simulink model "MR_CIGRE_RESISTIVO"  (R2017b)
settings: Solver=ode23tb  StartTime=0.0  StopTime=t_sim  RelTol=1e-4
values from neighbouring files (symbols this model uses):
  Cdc_Bat1 = 2E-3    (= 0.002)    [Dados_de_Bat_1.m]
  Cf_Bat1 = 5E-6    (= 5e-06)    [Dados_de_Bat_1.m]
  I_max_Bat1 = 1.5*Is_bat1*sqrt(2)    [Dados_de_Bat_1.m]
  Is_bat1 = Sb_Bat1 / (sqrt(3)*Vs2)    [Dados_de_Bat_1.m]
  K_iff_Bat1 = 0    [Dados_de_Bat_1.m]
  Kcij = Rfsj*(2*sig*w_ij*(Tpj + Tfsj)-1)    (= 3.9715)    [Dados_de_Bat_1.m]
  Ki_Bat1 = (R_Bat1+ron_Bat1)/ti_Bat1    (= 201.76)    [Dados_de_Bat_1.m]
  Kp_Bat1 = L_Bat1/ti_Bat1    (= 2.7)    [Dados_de_Bat_1.m]
  Kv_Bat1 = 0.75    [Dados_de_Bat_1.m]
  Kvi_DC = 25*Kvp_DC    (= 7.5)    [Dados_de_Bat_1.m]
  Kvp_DC = 0.3    [Dados_de_Bat_1.m]
  L_10_18 = imag(ug3)*C_10_18    [Dados_de_Linhas.m]
  L_12_13 = imag(ug3)*C_12_13    [Dados_de_Linhas.m]
  L_13_14 = imag(ug3)*C_13_14    [Dados_de_Linhas.m]
  L_14_15 = imag(ug3)*C_14_15    [Dados_de_Linhas.m]
  L_1_2 = imag(ug1)*C_1_2    [Dados_de_Linhas.m]
  L_2_3 = imag(ug1)*C_2_3    [Dados_de_Linhas.m]
  L_3_11 = imag(ug3)*C_3_11    [Dados_de_Linhas.m]
  L_3_4 = imag(ug1)*C_3_4    [Dados_de_Linhas.m]
  L_4_12 = imag(ug3)*C_4_12    [Dados_de_Linhas.m]
  L_4_5 = imag(ug1)*C_4_5    [Dados_de_Linhas.m]
  L_5_6 = imag(ug1)*C_5_6    [Dados_de_Linhas.m]
  L_6_16 = imag(ug3)*C_6_16    [Dados_de_Linhas.m]
  L_6_7 = imag(ug1)*C_6_7    [Dados_de_Linhas.m]
  L_7_8 = imag(ug1)*C_7_8    [Dados_de_Linhas.m]
  L_8_9 = imag(ug1)*C_8_9    [Dados_de_Linhas.m]
  L_9_10 = imag(ug1)*C_9_10    [Dados_de_Linhas.m]
  L_9_17 = imag(ug3)*C_9_17    [Dados_de_Linhas.m]
  L_Bat1 = 1.35E-3    (= 0.00135)    [Dados_de_Bat_1.m]
  L_Bat2 = 1.35E-3    (= 0.00135)    [Dados_de_Bat_2.m]
  L_Virt_Bat1 = 3e-3    (= 0.003)    [Dados_de_Bat_1.m]
  L_Virt_Bat2 = 3.0E-3    (= 0.003)    [Dados_de_Bat_2.m]
  LC_Bat2 = 1e-16    [Dados_de_Bat_2.m]
  Lfsj = 4e-3    (= 0.004)    [Dados_de_Bat_1.m]
  LPF_Ci_Bat1 = 8000    [Dados_de_Bat_1.m]
  LPF_Ci_Bat2 = 5000    [Dados_de_Bat_2.m]
  LPF_Cv_Bat1 = 3000    [Dados_de_Bat_1.m]
  LPF_Q_Bat1 = 3*2*pi()    [Dados_de_Bat_1.m]
  m_Bat1 = 0.05    [Dados_de_Bat_1.m]
  n_Bat1 = 0.05    [Dados_de_Bat_1.m]
  PQ_ref_taxavar_bat1 = 0.5    [Dados_de_Bat_1.m]
  R_10_18 = real(ug3)*C_10_18    [Dados_de_Linhas.m]
  R_12_13 = real(ug3)*C_12_13    [Dados_de_Linhas.m]
  R_13_14 = real(ug3)*C_13_14    [Dados_de_Linhas.m]
  R_14_15 = real(ug3)*C_14_15    [Dados_de_Linhas.m]
  R_1_2 = real(ug1)*C_1_2    [Dados_de_Linhas.m]
  R_2_3 = real(ug1)*C_2_3    [Dados_de_Linhas.m]
  R_3_11 = real(ug3)*C_3_11    [Dados_de_Linhas.m]
  R_3_4 = real(ug1)*C_3_4    [Dados_de_Linhas.m]
  R_4_12 = real(ug3)*C_4_12    [Dados_de_Linhas.m]
  R_4_5 = real(ug1)*C_4_5    [Dados_de_Linhas.m]
  R_5_6 = real(ug1)*C_5_6    [Dados_de_Linhas.m]
  R_6_16 = real(ug3)*C_6_16    [Dados_de_Linhas.m]
  R_6_7 = real(ug1)*C_6_7    [Dados_de_Linhas.m]
  R_7_8 = real(ug1)*C_7_8    [Dados_de_Linhas.m]
  R_8_9 = real(ug1)*C_8_9    [Dados_de_Linhas.m]
  R_9_10 = real(ug1)*C_9_10    [Dados_de_Linhas.m]
  R_9_17 = real(ug3)*C_9_17    [Dados_de_Linhas.m]
  R_Bat1 = 0.1    [Dados_de_Bat_1.m]
  R_Virt_Bat1 = 0    [Dados_de_Bat_1.m]
  R_Virt_Bat2 = 0    [Dados_de_Bat_2.m]
  Rb_bat1 = (N_cell_serie * Rb_cell) / N_string_cell    (= 0.153333333333)    [Dados_de_Bat_1.m]
  RC_Bat2 = 1e-16    [Dados_de_Bat_2.m]
  Rfsj = 0.03    [Dados_de_Bat_1.m]
  ron_Bat1 = 0.88E-3    (= 0.00088)    [Dados_de_Bat_1.m]
  Vdc_Bat1 = 800    [Dados_de_Bat_1.m]
  Voc_bat1 = N_cell_serie * Voc_cell    (= 180)    [Dados_de_Bat_1.m]
  z_Bat1 = z_gk    [Dados_de_Bat_1.m]
undefined symbols (not defined in the file or in its folder): BAT1_CONT, BAT2_CONT, Cdc, Cf, cont_fre, cont_ten, f0, Imax_solar1, Imax_solar2, Ki_interm, Kie, Kiw, Kp_cp, Kp_cr, Kp_interm, Kpe, Kpw, L, LPF_P_Bat1, LPF_P_Interm, LPF_Vdc, P_Solar1, P_Solar2, PQ_ref_time_bat1, Pref_Bat1, Qref_Bat1, Qref_Solar, R, ron, Sb_Bat1, Sb_ger, Sb_sol1, Sb_sol2, t_atraso, t_CS_ini, TDR1, TDR11, TDR15, TDR16, TDR17, TDR18, ti_cp, ti_cr, tilha, TLR11, TLR15, TLR16, TLR17, TLR18, tsinc, Vdc, vref1, Vref_sec, Vs1, Vs2, w0, wref_sec
libraries: powerlib x158, powerlib_meascontrol x59, re_lib x2, simulink x1
(part 1 of 4)
Description:
  | Copyright 2008-2016 The MathWorks, Inc.
settings Model: FPTRunName=Active  SimulationMode=accelerator  ExtModeTrigMode=oneshot  ExtModeArmWhenConnect=off  ExtModeAutoUpdateStatusClock=off  Creator=MathWorks  LastModifiedBy=KDRF
settings SolverCC: ZeroCrossAlgorithm=Adaptive
settings DataIOCC: FinalStateName=MR_estab  InitialState=MR_estab  SaveCompleteFinalSimState=on  SaveFormat=Array  SignalLoggingSaveFormat=ModelDataLogs  SignalLoggingName=sigsOut  OutputTimes=[0:1/20:10]
settings OptimizationCC: BlockReduction=off  BooleanDataType=off  ExpressionDepthLimit=2147483647  InitFltsAndDblsToZero=on  EfficientMapNaN2IntZero=off  LifeSpan=inf
settings DebuggingCC: UnderspecifiedInitializationDetection=Classic  MergeDetectMultiDrivingBlocksExec=none  CheckExecutionContextPreStartOutputMsg=on  CheckExecutionContextRuntimeOutputMsg=on  SignalResolutionControl=TryResolveAllWithWarning  IgnoredZcDiagnostic=none  MultiTaskDSMMsg=warning  MultiTaskCondExecSysMsg=none  SigSpecEnsureSampleTimeMsg=none  FcnCallInpInsideContextMsg=warning  UnconnectedInputMsg=none  UnconnectedOutputMsg=none  UnconnectedLineMsg=none  StateNameClashWarn=warning  SFUnexpectedBacktrackingDiag=warning  SFNoUnconditionalDefaultTransitionDiag=warning  SFExecutionAtInitializationDiag=none
settings HardwareCC: ProdBitPerPointer=32  ProdBitPerSizeT=32  ProdBitPerPtrDiffT=32  ProdLargestAtomicFloat=None  ProdIntDivRoundTo=Undefined  ProdEndianess=Unspecified  ProdWordSize=32  ProdHWDeviceType=Specified  TargetBitPerPointer=64  TargetBitPerSizeT=64  TargetBitPerPtrDiffT=64  TargetLongLongMode=on  TargetIntDivRoundTo=Zero  TargetEndianess=LittleEndian  TargetWordSize=64  TargetHWDeviceType=MATLAB Host  ProdEqTarget=off
settings ModelReferenceCC: PropagateSignalLabelsOutOfModel=off
settings CodeAppCC: MaxIdLength=128
settings GRTTargetCC: TargetLangStandard=C89/C90 (ANSI)  CombineOutputUpdateFcns=off  GRTInterface=on
settings ConfigComp: CovMetricSettings=dw  CovHtmlReporting=on  CovSaveCumulativeToWorkspaceVar=on  CovSaveSingleToWorkspaceVar=on  CovExternalEMLEnable=off  CovSFcnEnable=off
settings SimscapeCC: SimscapeNormalizeSystem=off

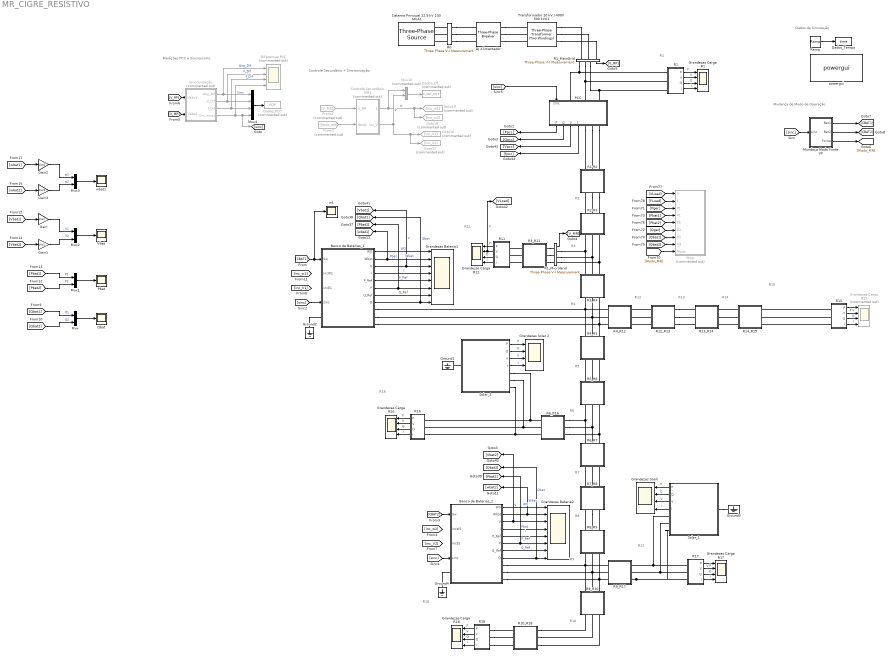
== system MR_CIGRE_RESISTIVO ==
  note: Medições PCC e Sincronismo
  note: Dados de Simulação
  note: R2
  note: R3
  note: R12
  note: R13
  note: R14
  note: R4
  note: R5
  note: R7
  note: R8
  note: R6
  note: R9
  note: R10
  note: R18
  note: R17
  note: R16
  note: R15
  note: R11
  note: R1
  note: Mudança de Modo de Operação
  note: Controle Secundário + Sincronização
  Banco de Baterias_1 : Subsystem
  Banco de Baterias_2 : Subsystem
  Controle Secundário MR1 : Subsystem  Commented=on
  "DJ Alimentador " : powerlib/Elements/Three-Phase Breaker  InitialState=closed  SwitchA=on  SwitchB=on  SwitchC=on  SwitchTimes=t_deslig_rede  External=off  BreakerResistance=0.01  SnubberResistance=1e5  SnubberCapacitance=inf  Measurements=None
      settings: AttributesFormatString=\n
  Dados_CS : ToWorkspace  Commented=on  VariableName=C_SEC_INC1  SaveFormat=Structure With Time  SampleTime=-1
  Dados_PCC : ToWorkspace  Commented=on  VariableName=PDF  SampleTime=-1
  Dados_Tempo : ToWorkspace  VariableName=time  SampleTime=-1
  Diferenças PCC : Scope  Commented=on  NumInputPorts=4
  From1 : From  Commented=on  GotoTag=Modo_MR
  From2 : From  Commented=on  GotoTag=V_MR
  Gain : Gain  Gain=1/Vs2
  Gain1 : Gain  Gain=1/Vs2
  Gain2 : Gain  Gain=1/w0
  Gain3 : Gain  Gain=1/w0
  Goto16 : Goto  Commented=on  GotoTag=inc_V1
  Goto17 : Goto  Commented=on  GotoTag=inc_V2
  Goto18 : Goto  Commented=on  GotoTag=inc_w2
  Goto19 : Goto  Commented=on  GotoTag=inc_w1
  Grandezas Bateria1 : Scope  NumInputPorts=8
  Grandezas Bateria2 : Scope  NumInputPorts=8
  Grandezas Carga R{1,11,16..18} (5 alike) : Scope  NumInputPorts=4
  Grandezas Carga R15 : Scope  Commented=on  NumInputPorts=4
  Grandezas Soalr : Scope  NumInputPorts=4
  Grandezas Solar 2 : Scope  NumInputPorts=4
  Ground{1..4} (4 alike) : powerlib/Elements/Ground  LConnTagsString=a
  Mundaça Modo Fonte VF : Subsystem
  Mux{,1..3} (4 alike) : Mux  Inputs=2
  Mux10 : Mux  Commented=on  Inputs=2
  Mux4 : Mux
  PCC : Subsystem
  Pbat : Scope
  Qbat : Scope
  R0 : powerlib/Measurements/Three-Phase V-I Measurement  VoltageMeasurement=phase-to-phase  SetLabelV=on  LabelV=V_sub  Vpu=off  VpuLL=off  CurrentMeasurement=no  SetLabelI=on  LabelI=Iabc_B120  Ipu=off  Pbase=100e6  Vbase=Vs1  OutputType=Complex  PhasorSimulation=on  PSBequivalent=0
  R1 : Subsystem
  R1-R2 : Subsystem
  R10_R18 : Subsystem
  R11 : Subsystem
  R12_R13 : Subsystem
  R13_R14 : Subsystem
  R14_R15 : Subsystem
  R15 : Subsystem
  R16 : Subsystem
  R17 : Subsystem
  R18 : Subsystem
  R1_MainGrid : powerlib/Measurements/Three-Phase V-I Measurement  VoltageMeasurement=phase-to-phase  SetLabelV=off  LabelV=Vabc_B120  Vpu=off  VpuLL=off  CurrentMeasurement=no  SetLabelI=off  LabelI=Iabc_B120  Ipu=off  Pbase=20e3  Vbase=Vs2  OutputType=Complex  PhasorSimulation=on  PSBequivalent=0
  R1_MicroGrid : powerlib/Measurements/Three-Phase V-I Measurement  VoltageMeasurement=phase-to-phase  SetLabelV=off  LabelV=Vabc_B120  Vpu=off  VpuLL=off  CurrentMeasurement=no  SetLabelI=off  LabelI=Iabc_B120  Ipu=off  Pbase=20e3  Vbase=Vs2  OutputType=Complex  PhasorSimulation=on  PSBequivalent=0
  R2-R3 : Subsystem
  R3_R11 : Subsystem
  R3_R4 : Subsystem
  R4_R12 : Subsystem
  R4_R5 : Subsystem
  R5_R6 : Subsystem
  R6_R16 : Subsystem
  R6_R7 : Subsystem
  R7_R8 : Subsystem
  R8_R9 : Subsystem
  R9_R10 : Subsystem
  R9_R17 : Subsystem
  Ramp : simulink/Sources/Ramp  slope=1  start=0  X0=0
  Sincronização : Subsystem  Commented=on
  Sistema Principal 22.9 kV 100 MVA1 : powerlib/Electrical Sources/Three-Phase Source  InternalConnection=Yg  VoltagePhases=off  Voltage=Vs1*vref1  PhaseAngle=0  Voltage_phases=[25e3 25e3 25e3]/sqrt(3)  PhaseAngles_phases=[0 -120 +120]  Frequency=f0  NonIdealSource=on  SpecifyImpedance=on  Resistance=25^2/1000/10  Inductance=25^2/1000/377  ShortCircuitLevel=100e6  BaseVoltage=Vs1  XRratio=1  BusType=swing  Pref=0  Qref=0  Prefabc=[10e3, 10e3, 10e3]  Qrefabc=[0, 0, 0]  Qmin=-Inf  Qmax=Inf
  Solar_1 : Subsystem
  Solar_2 : Subsystem
  Stop : Subsystem  Commented=on
  Transformador 20 kV / 400V 500 kVA1 : powerlib/Elements/Three-Phase Transformer (Two Windings)  Winding1Connection=Y  Winding2Connection=Yg  CoreType=Three single-phase transformers  SetSaturation=off  Hysteresis=off  DataFile='hysteresis'  SetInitialFlux=off  Measurements=None  UNITS=pu  NominalPower=[ 500e3 , 50 ]  Winding1=[Vs1 , 0.005 , 0.02]  Winding2=[Vs2 , 0.005 , 0.02 ]  Rm=200  Lm=200  L0=0.5  Saturation="[ 0,0  ;  0.005,1.2  ;  1.0,1.4 ]"  InitialFluxes=[ 0.8 , -0.8 , 0.7 ]  MoreParameters=off  BreakLoop=off  DataType=off  TransfoNumber=0
  Vbat : Scope
  powergui : powerlib/powergui  Priority=2  SimulationMode=Discrete  SampleTime=10e-6  frequency=60  Iterations=50  frequencyindice=0  Pbase=20e3  ErrMax=0.0001  UnitsV=V  UnitsW=kW  buscounter=0  FunctionMessages=off  echomessages=off  EnableUseOfTLC=off  CurrentSourceSwitches=off  DisableSnubberDevices=on  DisableRonSwitches=off  DisableVfSwitches=off  DisplayEquations=off  SolverType=Tustin  Interpol=off  ExternalGateDelay=off  methode=off  Ts=0  x0status=blocks  SPID=on  SwTol=0  HookPort=off  RestoreLinks=warning  ResistiveCurrentMeasurement=off  Frange=logspace(0,3,50)  Ylog=off  Xlog=off  ShowGrid=off  save=off  variable=ZData  structure=0  ZoomFFT=on  StartTime=0.0  cycles=2  DisplayStyle=off  fundamental=60  FreqAxis=off  MaxFrequency=1000  frequencyindicesteady=1  RmsSteady=1  display=off
  w1 : Scope
  wbat1 : Scope
  wires:
  Mux4/1 -> Dados_PCC/1
  Ramp/1 -> Dados_Tempo/1
  [V_MR] -> Sincronização/2(Vabc2)
  [V_RP] -> Sincronização/1(Vabc1)
  Sincronização/1(Ang_Dif) -> Diferenças PCC/1, Mux4/1  "Ang_Dif"
  Sincronização/2(V_Dif) -> Diferenças PCC/2, Mux4/2  "V_Dif"
  Sincronização/3(f_Dif) -> Diferenças PCC/3, Mux4/3  "f_Dif"
  Sincronização/4(Sinal sinc1) -> Diferenças PCC/4, [sinc], Mux4/4  "Sinc"
  Solar_2/1(P) -> Grandezas Solar 2/1  "P"
  Solar_2/2(Q) -> Grandezas Solar 2/2  "Q"
  Solar_2/3(V) -> Grandezas Solar 2/3  "V"
  Solar_2/4(I) -> Grandezas Solar 2/4  "I"
  Solar_1/1(P) -> Grandezas Soalr/1  "P"
  Solar_1/2(Q) -> Grandezas Soalr/2  "Q"
  Solar_1/3(V) -> Grandezas Soalr/3  "V"
  Solar_1/4(I) -> Grandezas Soalr/4  "I"
  R1_MainGrid/1 -> [V_RP]
  Banco de Baterias_1/2(Wbat) -> [wbat1], Grandezas Bateria1/2  "Wbat"
  Banco de Baterias_1/4(I) -> Grandezas Bateria1/4  "I"
  Banco de Baterias_1/7(Q_Ref) -> Grandezas Bateria1/7  "Q_Ref"
  Banco de Baterias_1/5(P_Ref) -> Grandezas Bateria1/5  "P_Ref"
  Banco de Baterias_1/3(V) -> [Vbat1], Grandezas Bateria1/3  "V"
  [CBAT1] -> w1/1, Banco de Baterias_1/1(Sw)
  Banco de Baterias_1/6(P) -> [Pbat1], Grandezas Bateria1/6  "Pbat"
  Banco de Baterias_1/8(Q) -> [Qbat1], Grandezas Bateria1/8  "Qbat"
  [sinc] -> Banco de Baterias_1/4(sinc)
  Banco de Baterias_1/1(W0) -> Grandezas Bateria1/1  "W0"
  Banco de Baterias_2/7(Q_Ref) -> Grandezas Bateria2/7  "Q_Ref"
  Banco de Baterias_2/6(P) -> [Pbat2], Grandezas Bateria2/6  "Pbat"
  Banco de Baterias_2/4(I) -> Grandezas Bateria2/4  "I"
  Banco de Baterias_2/8(Q) -> [Qbat2], Grandezas Bateria2/8  "Qbat"
  Banco de Baterias_2/3(V) -> [Vbat2], Grandezas Bateria2/3  "V"
  Banco de Baterias_2/1(W0) -> Grandezas Bateria2/1  "W0"
  [sinc] -> Banco de Baterias_2/4(sinc)
  [CBAT2] -> Banco de Baterias_2/1(Sw)
  Banco de Baterias_2/2(Wbat) -> [wbat2], Grandezas Bateria2/2  "Wbat"
  Banco de Baterias_2/5(P_Ref) -> Grandezas Bateria2/5  "P_Ref"
  R1_MicroGrid/1 -> [V_MR]
  [Pbat1] -> Stop/4(P2)
  [VLoad] -> Stop/1(V)
  [Qger] -> Stop/6(Q1)
  [Modo_MR] -> Stop/9(Modo)
  [Qbat1] -> Stop/7(Q2)
  [Pger] -> Stop/3(P1)
  [Qbat2] -> Stop/8(Q3)
  [FLoad] -> Stop/2(f)
  [Pbat2] -> Stop/5(P3)
  R11/1(P) -> Grandezas Carga R11/1  "P"
  R11/2(V) -> [VLoad], Grandezas Carga R11/2  "V"
  R11/3(Q) -> Grandezas Carga R11/3  "Q"
  R11/4(I) -> Grandezas Carga R11/4  "I"
  R15/3(Q) -> Grandezas Carga R15/3  "Q"
  R15/2(V) -> Grandezas Carga R15/2  "V"
  R15/4(I) -> Grandezas Carga R15/4  "I"
  R15/1(P) -> Grandezas Carga R15/1  "P"
  R16/4(I) -> Grandezas Carga R16/4  "I"
  R16/3(Q) -> Grandezas Carga R16/3  "Q"
  R16/2(V) -> Grandezas Carga R16/2  "V"
  R16/1(P) -> Grandezas Carga R16/1  "P"
  R17/1(P) -> Grandezas Carga R17/1  "P"
  R17/3(Q) -> Grandezas Carga R17/3  "Q"
  R17/4(I) -> Grandezas Carga R17/4  "I"
  R17/2(V) -> Grandezas Carga R17/2  "V"
  R18/3(Q) -> Grandezas Carga R18/3  "Q"
  R18/2(V) -> Grandezas Carga R18/2  "V"
  R18/4(I) -> Grandezas Carga R18/4  "I"
  R18/1(P) -> Grandezas Carga R18/1  "P"
  R1/2(V) -> Grandezas Carga R1/2  "V"
  R1/4(I) -> Grandezas Carga R1/4  "I"
  R1/3(Q) -> Grandezas Carga R1/3  "Q"
  R1/1(P) -> Grandezas Carga R1/1  "P"
  PCC/4(f) -> [fpcc]
  PCC/3(V) -> [Vpcc]
  PCC/2(Q) -> [Qpcc]
  PCC/1(P) -> [Ppcc]
  [sinc] -> PCC/1(sinc)
  Mundaça Modo Fonte VF/1(Bat1) -> [CBAT1]
  Mundaça Modo Fonte VF/3(Fonte) -> [Modo_MR]
  Mundaça Modo Fonte VF/2(Bat2) -> [CBAT2]
  [sinc] -> Mundaça Modo Fonte VF/1(sinc)
  Controle Secundário MR1/1(Inc_w) -> Goto18/1, Goto19/1, Mux10/1  "w"
  Mux10/1 -> Dados_CS/1
  From2/1 -> Controle Secundário MR1/1(V_MR)
  From1/1 -> Controle Secundário MR1/2(Modo)
  Controle Secundário MR1/2(Inc_V) -> Goto17/1, Goto16/1, Mux10/2  "V"
  Mux/1 -> Qbat/1
  [Qbat1] -> Mux/1  "Q1"
  [Qbat2] -> Mux/2  "Q2"
  [Pbat1] -> Mux1/1  "P1"
  Mux1/1 -> Pbat/1
  [Pbat2] -> Mux1/2  "P2"
  [Vbat2] -> Gain1/1
  Mux2/1 -> Vbat/1
  [Vbat1] -> Gain/1
  Gain/1 -> Mux2/1  "V1"
  Gain1/1 -> Mux2/2  "V2"
  Mux3/1 -> wbat1/1
  Gain2/1 -> Mux3/1  "w1"
  [wbat1] -> Gain2/1
  Gain3/1 -> Mux3/2  "w2"
  [wbat2] -> Gain3/1
  connections:
  Solar_2/LConn1 -- Ground1/LConn1
  Solar_1/LConn1 -- Ground3/LConn1
  R3_R4/RConn1 -- R1_MicroGrid/RConn1 -- R2-R3/RConn1
  R3_R4/RConn2 -- R1_MicroGrid/RConn2 -- R2-R3/RConn2
  R3_R4/RConn3 -- R1_MicroGrid/RConn3 -- R2-R3/RConn3
  R12_R13/LConn1 -- R4_R12/RConn1
  R12_R13/LConn2 -- R4_R12/RConn2
  R12_R13/LConn3 -- R4_R12/RConn3
  R4_R12/LConn1 -- Banco de Baterias_1/RConn1 -- R4_R5/LConn1 -- R3_R4/LConn1
  R4_R12/LConn2 -- Banco de Baterias_1/RConn2 -- R4_R5/LConn2 -- R3_R4/LConn2
  R4_R12/LConn3 -- Banco de Baterias_1/RConn3 -- R4_R5/LConn3 -- R3_R4/LConn3
  R14_R15/LConn3 -- R13_R14/RConn3
  R14_R15/LConn1 -- R13_R14/RConn1
  R14_R15/LConn2 -- R13_R14/RConn2
  R12_R13/RConn1 -- R13_R14/LConn1
  R12_R13/RConn2 -- R13_R14/LConn2
  R12_R13/RConn3 -- R13_R14/LConn3
  R15/LConn1 -- R14_R15/RConn1
  R15/LConn2 -- R14_R15/RConn2
  R15/LConn3 -- R14_R15/RConn3
  R5_R6/LConn1 -- R4_R5/RConn1
  R5_R6/LConn2 -- R4_R5/RConn2
  R5_R6/LConn3 -- R4_R5/RConn3
  R16/LConn1 -- Solar_2/RConn1 -- R6_R16/RConn1
  R16/LConn3 -- Solar_2/RConn3 -- R6_R16/RConn3
  R16/LConn2 -- Solar_2/RConn2 -- R6_R16/RConn2
  R6_R16/LConn1 -- R6_R7/LConn1 -- R5_R6/RConn1
  R6_R16/LConn2 -- R6_R7/LConn2 -- R5_R6/RConn2
  R6_R16/LConn3 -- R6_R7/LConn3 -- R5_R6/RConn3
  R7_R8/LConn2 -- R6_R7/RConn2
  R7_R8/LConn1 -- R6_R7/RConn1
  R7_R8/LConn3 -- R6_R7/RConn3
  R8_R9/LConn1 -- R7_R8/RConn1
  R8_R9/LConn3 -- R7_R8/RConn3
  R7_R8/RConn2 -- R8_R9/LConn2
  R17/LConn1 -- Solar_1/RConn1 -- R9_R17/RConn1
  R17/LConn2 -- Solar_1/RConn2 -- R9_R17/RConn2
  R9_R17/RConn3 -- Solar_1/RConn3 -- R17/LConn3
  R9_R17/LConn1 -- Banco de Baterias_2/RConn1 -- R9_R10/LConn1 -- R8_R9/RConn1
  R9_R17/LConn2 -- Banco de Baterias_2/RConn2 -- R9_R10/LConn2 -- R8_R9/RConn2
  R9_R17/LConn3 -- Banco de Baterias_2/RConn3 -- R9_R10/LConn3 -- R8_R9/RConn3
  R10_R18/LConn1 -- R9_R10/RConn1
  R10_R18/LConn2 -- R9_R10/RConn2
  R10_R18/LConn3 -- R9_R10/RConn3
  R0/RConn1 -- Sistema Principal 22.9 kV 100 MVA1/RConn3
  R0/RConn2 -- Sistema Principal 22.9 kV 100 MVA1/RConn2
  R0/RConn3 -- Sistema Principal 22.9 kV 100 MVA1/RConn1
  R0/LConn1 -- "DJ Alimentador "/RConn3
  R0/LConn2 -- "DJ Alimentador "/RConn2
  R0/LConn3 -- "DJ Alimentador "/RConn1
  Transformador 20 kV / 400V 500 kVA1/RConn1 -- R1_MainGrid/LConn3
  Transformador 20 kV / 400V 500 kVA1/RConn2 -- R1_MainGrid/LConn2
  Transformador 20 kV / 400V 500 kVA1/RConn3 -- R1_MainGrid/LConn1
  PCC/RConn1 -- R1-R2/LConn1
  R1-R2/RConn1 -- R2-R3/LConn1
  R1-R2/RConn2 -- R2-R3/LConn2
  R1-R2/RConn3 -- R2-R3/LConn3
  Banco de Baterias_1/LConn1 -- Ground2/LConn1
  Banco de Baterias_2/LConn1 -- Ground4/LConn1
  R3_R11/LConn1 -- R1_MicroGrid/LConn1
  R3_R11/LConn2 -- R1_MicroGrid/LConn2
  R3_R11/LConn3 -- R1_MicroGrid/LConn3
  R3_R11/RConn1 -- R11/LConn1
  R3_R11/RConn3 -- R11/LConn3
  R3_R11/RConn2 -- R11/LConn2
  R18/LConn1 -- R10_R18/RConn1
  R18/LConn2 -- R10_R18/RConn2
  R18/LConn3 -- R10_R18/RConn3
  PCC/RConn2 -- R1-R2/LConn2
  PCC/RConn3 -- R1-R2/LConn3
  R1_MainGrid/RConn2 -- R1/LConn2 -- PCC/LConn2
  R1_MainGrid/RConn3 -- R1/LConn1 -- PCC/LConn1
  R1_MainGrid/RConn1 -- R1/LConn3 -- PCC/LConn3
  "DJ Alimentador "/LConn1 -- Transformador 20 kV / 400V 500 kVA1/LConn1
  "DJ Alimentador "/LConn2 -- Transformador 20 kV / 400V 500 kVA1/LConn2
  "DJ Alimentador "/LConn3 -- Transformador 20 kV / 400V 500 kVA1/LConn3

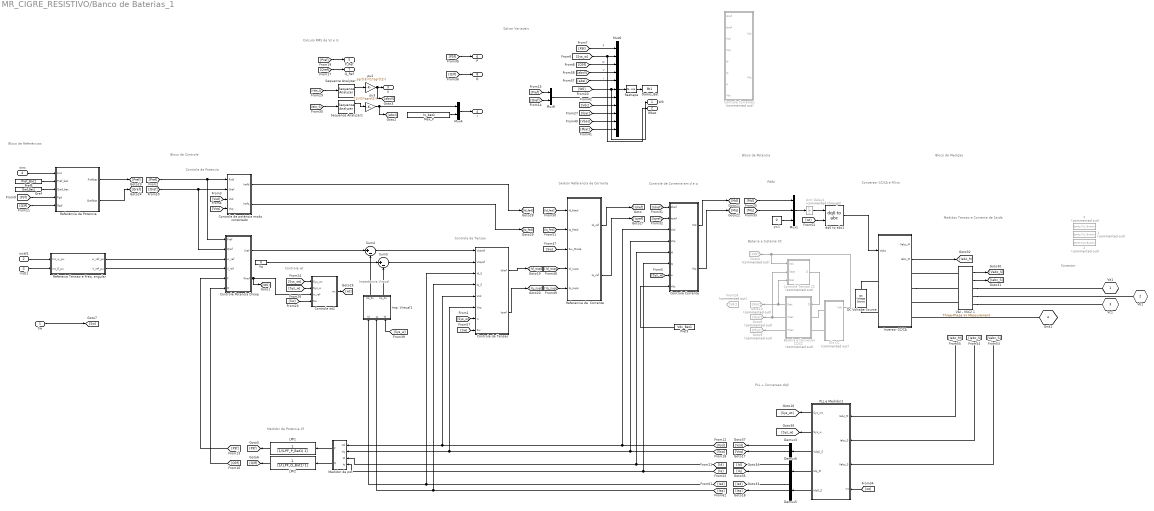
== system MR_CIGRE_RESISTIVO/Banco de Baterias_1 ==
  note: Bloco de Controle
  note: Controle de Corrente
      | em d e q
  note: Calculo RMS de Vs e Is
  note: Medidor de Potência 3f
  note: Seletor Referencia
      |      de Corrente
  note: Controle de Tensao
  note: Impedancia
      | 					  Virtual
  note: PWM
  note: Conversor CC/CA
      |           e Filtro
  note: Bloco de Potencia
  note: Bloco de Mediçao
  note: Medidas Tensao e
      |    Corrente de Saida
  note: PLL + Conversao dq0
  note: Bloco de Referências
  note: Controle de Potencia
  note: Controle wt
  note: Conector
  note: Bateria e Sistema CC
  note: Salvar Variaveis
  Sw : Inport
  incW1 : Inport  Port=2
  incE1 : Inport  Port=3
  sinc : Inport  Port=4
  1 : powerlib/Elements/Series RLC Branch  Commented=on  LConnTagsString=__new0  RConnTagsString=__new0  BranchType=RL  Resistance=RC_Bat2  Inductance=LC_Bat2  SetiL0=off  InitialCurrent=0  Capacitance=1e-6  Setx0=off  InitialVoltage=0  Measurements=None
  2 : powerlib/Elements/Series RLC Branch  Commented=on  LConnTagsString=__new0  RConnTagsString=__new0  BranchType=RL  Resistance=RC_Bat2  Inductance=LC_Bat2  SetiL0=off  InitialCurrent=0  Capacitance=1e-6  Setx0=off  InitialVoltage=0  Measurements=None
  9 : powerlib/Elements/Series RLC Branch  Commented=on  LConnTagsString=__new0  RConnTagsString=__new0  BranchType=RL  Resistance=RC_Bat2  Inductance=LC_Bat2  SetiL0=off  InitialCurrent=0  Capacitance=1e-6  Setx0=off  InitialVoltage=0  Measurements=None
  Bateria e Conversor CC/CC : Subsystem  Commented=on
  Controle Corrente : Subsystem
  Controle Corrente1 : Subsystem  Commented=on
  Controle Tensao CC : Subsystem  Commented=on
  Controle Potencia Droop : Subsystem
  Controle de Tensao : Subsystem
  Controle de potência modo conectado : Subsystem
  Controle wt2 : Subsystem
  DC Voltage Source : powerlib/Electrical Sources/DC Voltage Source  Amplitude=Vdc_Bat1  Measurements=None
  Dados_Bat : ToWorkspace  VariableName=Bt1  SaveFormat=Structure With Time  SampleTime=-1
  Demux3 : Demux  Outputs=3
  Demux5 : Demux  Outputs=3
  Demux6 : Demux  Outputs=3
  Elo CC : Subsystem  Commented=on
  From28 : From  Commented=on  GotoTag=Vdc
  Goto10 : Goto  Commented=on  GotoTag=Ibat
  Goto4 : Goto  Commented=on  GotoTag=Vdc
  Goto8 : Goto  Commented=on  GotoTag=Vbat
  Goto9 : Goto  Commented=on  GotoTag=Pbat
  Imp. Virtual1 : Subsystem
  Inversor CC/CA : Subsystem
  LPF1 : TransferFcn  Denominator=[1/(LPF_P_Bat1) 1]
  LPF2 : TransferFcn  Denominator=[1/(LPF_Q_Bat1) 1]
  Max_P : Constant  Value=Is_bat1
  Medidor de pot : Subsystem
  Mux1 : Mux  Inputs=3
  Mux4 : Mux  Inputs=2
  Mux6 : Mux  Inputs=11
  Mux8 : Mux  Inputs=2
  PLL e Medidor1 : Subsystem
  Pref3 : Constant  Value=Vdc_Bat1
  Pref5 : Constant  Value=Pref_Bat1
  Qref : Constant  Value=Qref_Bat1
  Referecia Tensao e Freq. angular : Subsystem
  Referencia de  Corrente : Subsystem
  Referência de Potencia : Subsystem
  Reshape : Reshape  OutputDimensions=[1,7]
  Sequence Analyzer : powerlib_meascontrol/Measurements/Sequence Analyzer  Freq=f0  n=1  seq=Positive  InInit=[1, 0]  Ts=0
      settings: SourceProductName=Simscape Power Systems  SourceProductBaseCode=PS
  Sequence Analyzer1 : powerlib_meascontrol/Measurements/Sequence Analyzer  Freq=f0  n=1  seq=Positive  InInit=[1, 0]  Ts=0
      settings: SourceProductName=Simscape Power Systems  SourceProductBaseCode=PS
  Sum4 : Sum  Inputs=|+-
  Sum5 : Sum  Inputs=|+-
  Unit Delay1 : UnitDelay  Commented=through  SampleTime=5E-6
  V&I - VSC2 1 : powerlib/Measurements/Three-Phase V-I Measurement  VoltageMeasurement=phase-to-ground  SetLabelV=off  LabelV=Vabc  Vpu=off  VpuLL=off  CurrentMeasurement=yes  SetLabelI=off  LabelI=Iabc  Ipu=off  Pbase=100e6  Vbase=500e3  OutputType=Complex  PhasorSimulation=off  PSBequivalent=0
  Vq : Constant  Value=0
  dq0 to abc1 : powerlib_meascontrol/Transformations/dq0 to abc  Alignment=90 degrees behind phase A axis
  pu2 : Gain  Gain=sqrt(3)/(1*sqrt(2))
  pu3 : Gain  Gain=(1)/(1*sqrt(2))
  y=1 : Constant  Value=0
  Va1 : PMIOPort  Port=1  Side=Right
  Vb1 : PMIOPort  Port=2  Side=Right
  Vc1 : PMIOPort  Port=3  Side=Right
  Gnd1 : PMIOPort  Port=4  Side=Left
  W0 : Outport
  Wbat : Outport  Port=2
  V : Outport  Port=3
  I : Outport  Port=4
  P_Ref : Outport  Port=5
  P : Outport  Port=6
  Q_Ref : Outport  Port=7
  Q : Outport  Port=8
  wires:
  Sequence Analyzer/1 -> pu2/1
  pu2/1 -> [absV], V/1
  Sequence Analyzer1/1 -> pu3/1
  [Vabc_S] -> Sequence Analyzer/1
  [Iabc_S] -> Sequence Analyzer1/1
  [Sys_w] -> Controle Corrente/7(w)
  [Iq] -> Medidor de pot/4(Iq), Controle Corrente/6(Iq)
  [Idref] -> Controle Corrente/1(Idref)
  [Iqref] -> Controle Corrente/2(Iqref)
  Controle Corrente/1(Md) -> [Md]
  Mux4/1 -> I/1
  pu3/1 -> Mux4/1, [absI]
  [Q3f] -> Q/1
  Max_P/1 -> Mux4/2
  Referencia de  Corrente/1(Id_ref) -> [Idref]
  [Sw] -> Referencia de  Corrente/3(Sw_Mode)
  Controle de Tensao/1(Idref) -> [Id_sup]
  Controle de Tensao/2(Iqref) -> [Iq_sup]
  [Iq_sup] -> Referencia de  Corrente/5(Iq_supp)
  [Id_fed] -> Referencia de  Corrente/1(Id_feed)
  [Iq_fed] -> Referencia de  Corrente/2(Iq_feed)
  Controle de potência modo conectado/1(Irefd) -> [Id_fed]
  Controle de potência modo conectado/2(Irefq) -> [Iq_fed]
  [Mq] -> Mux1/2
  [Md] -> Mux1/1
  V&I - VSC2 1/2 -> [Iabc_S]
  V&I - VSC2 1/1 -> [Vabc_S]
  Mux1/1 -> Unit Delay1/1
  y=1/1 -> Mux1/3
  Inversor CC/CA/2(Iabc_M) -> [Iabc_M]
  Sum4/1 -> Controle de Tensao/1(Vsdref)
  Sum5/1 -> Controle de Tensao/2(Vsqref)
  Demux6/1 -> [Id]
  [wt] -> PLL e Medidor1/4(wt)
  PLL e Medidor1/5(Idq0_S) -> Demux5/1
  PLL e Medidor1/4(Idq_M) -> Demux6/1
  PLL e Medidor1/3(Vdq0_S) -> Demux3/1
  Demux5/1 -> [Isd]
  Demux6/2 -> [Iq]
  PLL e Medidor1/2(Sys_w) -> [Sys_w]
  Demux3/1 -> [Vsd]
  PLL e Medidor1/1(Sys_wt) -> [Sys_wt]
  Demux5/2 -> [Isq]
  Demux3/2 -> [Vsq]
  [Sw] -> Controle de Tensao/8(Sw)
  [Sys_w] -> Controle de Tensao/7(w)
  [Isq] -> Controle de Tensao/4(Iq_S), Imp. Virtual1/2(Iq)
  [Isd] -> Controle de Tensao/3(Id_S), Imp. Virtual1/1(Id)
  Sw/1 -> [Sw]
  Referência de Potencia/2(Qrefbat) -> [Qref]
  incE1/1 -> Referecia Tensao e Freq. angular/2(Inc_E_pu)
  Pref5/1 -> Referência de Potencia/2(Pref_bat)
  [P3f] -> Referência de Potencia/4(Pgd)
  Qref/1 -> Referência de Potencia/3(Qref_bat)
  [Q3f] -> Referência de Potencia/5(Qgd)
  Referência de Potencia/1(Prefbat) -> [Pref]
  sinc/1 -> Referência de Potencia/1(sinc)
  incW1/1 -> Referecia Tensao e Freq. angular/1(Inc_w_pu)
  [Pref] -> Controle Potencia Droop/1(Pref), Controle de potência modo conectado/1(Pref)
  [Qref] -> Controle Potencia Droop/2(Qref), Controle de potência modo conectado/2(Qref)
  Referecia Tensao e Freq. angular/1(w_ref_pu) -> Controle Potencia Droop/3(w_ref)
  Referecia Tensao e Freq. angular/2(V_ref_pu) -> Controle Potencia Droop/4(V_ref)
  [P3f] -> Controle Potencia Droop/5(P)
  [Q3f] -> Controle Potencia Droop/6(Q)
  Vq/1 -> Sum5/1
  [Pref] -> P_Ref/1
  [Qref] -> Q_Ref/1
  [P3f] -> P/1
  [Sys_w] -> Imp. Virtual1/3(W)
  [Sw] -> Controle wt2/4(Sw)
  [Sys_wt] -> Controle wt2/1(Sys_wt)
  Controle Potencia Droop/2(Wref) -> Controle wt2/3(w_ref), [W0]
  [Vsd] -> Controle de potência modo conectado/3(Vsd)
  [Vsq] -> Controle de potência modo conectado/4(Vsq)
  [Sys_w] -> Controle wt2/2(Sys_w)
  LPF1/1 -> [P3f]
  LPF2/1 -> [Q3f]
  Medidor de pot/2(Q) -> LPF2/1
  [Iabc_M] -> PLL e Medidor1/1(Iabc_M)
  [Iabc_S] -> PLL e Medidor1/2(Iabc_S)
  Controle Potencia Droop/1(Vref) -> Sum4/1
  Imp. Virtual1/1(Vd_Zv) -> Sum4/2
  Imp. Virtual1/2(Vq_Zv) -> Sum5/2
  Controle wt2/1(wt) -> [wt]
  [wt] -> dq0 to abc1/2
  dq0 to abc1/1 -> Inversor CC/CA/1(Vabc)
  Referencia de  Corrente/2(Iq_ref) -> [Iqref]
  [Id_sup] -> Referencia de  Corrente/4(Id_supp)
  [Id] -> Medidor de pot/3(Id), Controle Corrente/5(Id)
  [Vabc_S] -> PLL e Medidor1/3(Vabc_S)
  [Vsd] -> Controle de Tensao/5(Vsd), Medidor de pot/1(Vd), Controle Corrente/3(Vsd)
  [Vsq] -> Medidor de pot/2(Vq), Controle de Tensao/6(Vsq), Controle Corrente/4(Vsq)
  Controle Corrente/2(Mq) -> [Mq]
  Medidor de pot/1(P) -> LPF1/1
  Bateria e Conversor CC/CC/1(Ibat) -> Goto10/1, Controle Tensao CC/3(Ibat)
  Controle Tensao CC/1(D) -> Bateria e Conversor CC/CC/1(D)
  Bateria e Conversor CC/CC/3(Pbat) -> Goto9/1
  Bateria e Conversor CC/CC/2(Vbat) -> Goto8/1, Controle Tensao CC/2(Vbat)
  Elo CC/1(Vdc) -> Controle Tensao CC/1(Vdc), Goto4/1
  [Q3f] -> Mux6/3  "Q"
  [W0] -> W0/1, Mux6/6
  Mux8/1 -> Mux6/7
  Mux6/1 -> Reshape/1
  Reshape/1 -> Dados_Bat/1
  [absV] -> Mux6/4  "V"
  [Pbat] -> Mux6/11
  [P3f] -> Mux6/1  "P"
  [absI] -> Mux6/5  "I"
  [Vbat] -> Mux6/10
  [Vdc] -> Mux6/8
  [Pref] -> Mux8/1
  [Sys_w] -> Wbat/1, Mux6/2
  [Qref] -> Mux8/2
  [Ibat] -> Mux6/9
  Unit Delay1/1 -> dq0 to abc1/1
  Pref3/1 -> Controle Corrente/8(Vdc)
  connections:
  Gnd1/RConn1 -- Inversor CC/CA/RConn4
  V&I - VSC2 1/RConn3 -- Vc1/RConn1
  Inversor CC/CA/RConn2 -- V&I - VSC2 1/LConn2
  V&I - VSC2 1/RConn1 -- Va1/RConn1
  V&I - VSC2 1/LConn1 -- Inversor CC/CA/RConn1
  V&I - VSC2 1/LConn3 -- Inversor CC/CA/RConn3
  V&I - VSC2 1/RConn2 -- Vb1/RConn1
  Elo CC/LConn1 -- Bateria e Conversor CC/CC/LConn1
  Elo CC/LConn2 -- Bateria e Conversor CC/CC/LConn2
  DC Voltage Source/RConn1 -- Inversor CC/CA/LConn1
  DC Voltage Source/LConn1 -- Inversor CC/CA/LConn2

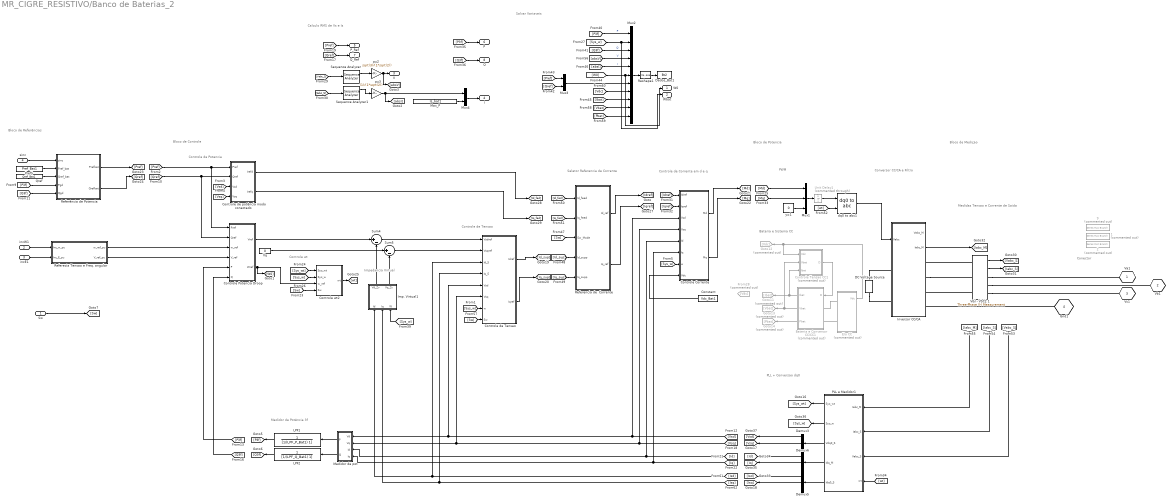
== system MR_CIGRE_RESISTIVO/Banco de Baterias_2 ==
  note: Bloco de Controle
  note: Controle de Corrente
      | em d e q
  note: Calculo RMS de Vs e Is
  note: Medidor de Potência 3f
  note: Seletor Referencia
      |      de Corrente
  note: Controle de Tensao
  note: Impedancia
      | 					  Virtual
  note: PWM
  note: Conversor CC/CA
      |           e Filtro
  note: Bloco de Potencia
  note: Bloco de Mediçao
  note: Medidas Tensao e
      |    Corrente de Saida
  note: PLL + Conversao dq0
  note: Bloco de Referências
  note: Controle de Potencia
  note: Controle wt
  note: Conector
  note: Salvar Variaveis
  note: Bateria e Sistema CC
  Sw : Inport
  incW1 : Inport  Port=2
  incE1 : Inport  Port=3
  sinc : Inport  Port=4
  1 : powerlib/Elements/Series RLC Branch  Commented=on  LConnTagsString=__new0  RConnTagsString=__new0  BranchType=RL  Resistance=RC_Bat2  Inductance=LC_Bat2  SetiL0=off  InitialCurrent=0  Capacitance=1e-6  Setx0=off  InitialVoltage=0  Measurements=None
  2 : powerlib/Elements/Series RLC Branch  Commented=on  LConnTagsString=__new0  RConnTagsString=__new0  BranchType=RL  Resistance=RC_Bat2  Inductance=LC_Bat2  SetiL0=off  InitialCurrent=0  Capacitance=1e-6  Setx0=off  InitialVoltage=0  Measurements=None
  9 : powerlib/Elements/Series RLC Branch  Commented=on  LConnTagsString=__new0  RConnTagsString=__new0  BranchType=RL  Resistance=RC_Bat2  Inductance=LC_Bat2  SetiL0=off  InitialCurrent=0  Capacitance=1e-6  Setx0=off  InitialVoltage=0  Measurements=None
  Bateria e Conversor CC/CC1 : Subsystem  Commented=on
  Constant : Constant  Value=Vdc_Bat1
  Controle Corrente : Subsystem
  Controle Tensao CC1 : Subsystem  Commented=on
  Controle Potencia Droop : Subsystem
  Controle de Tensao : Subsystem
  Controle de potência modo conectado : Subsystem
  Controle wt2 : Subsystem
  DC Voltage Source : powerlib/Electrical Sources/DC Voltage Source  Amplitude=Vdc_Bat1  Measurements=None
  Dados_Bat1 : ToWorkspace  VariableName=Bt2  SaveFormat=Structure With Time  SampleTime=-1
  Demux3 : Demux  Outputs=3
  Demux5 : Demux  Outputs=3
  Demux6 : Demux  Outputs=3
  Elo CC : Subsystem  Commented=on
  From28 : From  Commented=on  GotoTag=Vdc
  Goto11 : Goto  Commented=on  GotoTag=Ibat
  Goto12 : Goto  Commented=on  GotoTag=Vdc
  Goto13 : Goto  Commented=on  GotoTag=Vbat
  Goto14 : Goto  Commented=on  GotoTag=Pbat
  Imp. Virtual1 : Subsystem
  Inversor CC/CA : Subsystem
  LPF1 : TransferFcn  Denominator=[1/(LPF_P_Bat1) 1]
  LPF2 : TransferFcn  Denominator=[1/(LPF_Q_Bat1) 1]
  Max_P : Constant  Value=Is_bat1
  Medidor de pot : Subsystem
  Mux1 : Mux  Inputs=3
  Mux2 : Mux  Inputs=11
  Mux3 : Mux  Inputs=2
  Mux4 : Mux  Inputs=2
  PLL e Medidor1 : Subsystem
  Pref5 : Constant  Value=Pref_Bat1
  Qref : Constant  Value=Qref_Bat1
  Referecia Tensao e Freq. angular : Subsystem
  Referencia de  Corrente : Subsystem
  Referência de Potencia : Subsystem
  Reshape1 : Reshape  OutputDimensions=[1,7]
  Sequence Analyzer : powerlib_meascontrol/Measurements/Sequence Analyzer  Freq=f0  n=1  seq=Positive  InInit=[1, 0]  Ts=0
      settings: SourceProductName=Simscape Power Systems  SourceProductBaseCode=PS
  Sequence Analyzer1 : powerlib_meascontrol/Measurements/Sequence Analyzer  Freq=f0  n=1  seq=Positive  InInit=[1, 0]  Ts=0
      settings: SourceProductName=Simscape Power Systems  SourceProductBaseCode=PS
  Sum4 : Sum  Inputs=|+-
  Sum5 : Sum  Inputs=|+-
  Unit Delay1 : UnitDelay  Commented=through  SampleTime=5E-6
  V&I - VSC2 1 : powerlib/Measurements/Three-Phase V-I Measurement  VoltageMeasurement=phase-to-ground  SetLabelV=off  LabelV=Vabc  Vpu=off  VpuLL=off  CurrentMeasurement=yes  SetLabelI=off  LabelI=Iabc  Ipu=off  Pbase=100e6  Vbase=500e3  OutputType=Complex  PhasorSimulation=off  PSBequivalent=0
  Vq : Constant  Value=0
  dq0 to abc1 : powerlib_meascontrol/Transformations/dq0 to abc  Alignment=90 degrees behind phase A axis
  pu2 : Gain  Gain=sqrt(3)/(1*sqrt(2))
  pu3 : Gain  Gain=(1)/(1*sqrt(2))
  y=1 : Constant  Value=0
  Va1 : PMIOPort  Port=1  Side=Right
  Vb1 : PMIOPort  Port=2  Side=Right
  Vc1 : PMIOPort  Port=3  Side=Right
  Gnd1 : PMIOPort  Port=4  Side=Left
  W0 : Outport
  Wbat : Outport  Port=2
  V : Outport  Port=3
  I : Outport  Port=4
  P_Ref : Outport  Port=5
  P : Outport  Port=6
  Q_Ref : Outport  Port=7
  Q : Outport  Port=8
  wires:
  Sequence Analyzer/1 -> pu2/1
  pu2/1 -> [absV], V/1
  Sequence Analyzer1/1 -> pu3/1
  [Vabc_S] -> Sequence Analyzer/1
  [Iabc_S] -> Sequence Analyzer1/1
  [Sys_w] -> Controle Corrente/7(w)
  [Iq] -> Controle Corrente/6(Iq), Medidor de pot/4(Iq)
  [Idref] -> Controle Corrente/1(Idref)
  [Iqref] -> Controle Corrente/2(Iqref)
  Controle Corrente/1(Md) -> [Md]
  Mux4/1 -> I/1
  pu3/1 -> Mux4/1, [absI]
  [Q3f] -> Q/1
  Max_P/1 -> Mux4/2
  Referencia de  Corrente/1(Id_ref) -> [Idref]
  [Sw] -> Referencia de  Corrente/3(Sw_Mode)
  Controle de Tensao/1(Idref) -> [Id_sup]
  Controle de Tensao/2(Iqref) -> [Iq_sup]
  [Iq_sup] -> Referencia de  Corrente/5(Iq_supp)
  [Id_fed] -> Referencia de  Corrente/1(Id_feed)
  [Iq_fed] -> Referencia de  Corrente/2(Iq_feed)
  Controle de potência modo conectado/1(Irefd) -> [Id_fed]
  Controle de potência modo conectado/2(Irefq) -> [Iq_fed]
  [Mq] -> Mux1/2
  [Md] -> Mux1/1
  V&I - VSC2 1/2 -> [Iabc_S]
  V&I - VSC2 1/1 -> [Vabc_S]
  Mux1/1 -> Unit Delay1/1
  y=1/1 -> Mux1/3
  Inversor CC/CA/2(Iabc_M) -> [Iabc_M]
  Sum4/1 -> Controle de Tensao/1(Vsdref)
  Sum5/1 -> Controle de Tensao/2(Vsqref)
  Demux6/1 -> [Id]
  [wt] -> PLL e Medidor1/4(wt)
  PLL e Medidor1/5(Idq0_S) -> Demux5/1
  PLL e Medidor1/4(Idq_M) -> Demux6/1
  PLL e Medidor1/3(Vdq0_S) -> Demux3/1
  Demux5/1 -> [Isd]
  Demux6/2 -> [Iq]
  PLL e Medidor1/2(Sys_w) -> [Sys_w]
  Demux3/1 -> [Vsd]
  PLL e Medidor1/1(Sys_wt) -> [Sys_wt]
  Demux5/2 -> [Isq]
  Demux3/2 -> [Vsq]
  [Sw] -> Controle de Tensao/8(Sw)
  [Sys_w] -> Controle de Tensao/7(w)
  [Isq] -> Controle de Tensao/4(Iq_S), Imp. Virtual1/2(Iq)
  [Isd] -> Controle de Tensao/3(Id_S), Imp. Virtual1/1(Id)
  Sw/1 -> [Sw]
  Referência de Potencia/2(Qrefbat) -> [Qref]
  incE1/1 -> Referecia Tensao e Freq. angular/2(Inc_E_pu)
  Pref5/1 -> Referência de Potencia/2(Pref_bat)
  [P3f] -> Referência de Potencia/4(Pgd)
  Qref/1 -> Referência de Potencia/3(Qref_bat)
  [Q3f] -> Referência de Potencia/5(Qgd)
  Referência de Potencia/1(Prefbat) -> [Pref]
  sinc/1 -> Referência de Potencia/1(sinc)
  incW1/1 -> Referecia Tensao e Freq. angular/1(Inc_w_pu)
  [Pref] -> Controle Potencia Droop/1(Pref), Controle de potência modo conectado/1(Pref)
  [Qref] -> Controle Potencia Droop/2(Qref), Controle de potência modo conectado/2(Qref)
  Referecia Tensao e Freq. angular/1(w_ref_pu) -> Controle Potencia Droop/3(w_ref)
  Referecia Tensao e Freq. angular/2(V_ref_pu) -> Controle Potencia Droop/4(V_ref)
  [P3f] -> Controle Potencia Droop/5(P)
  [Q3f] -> Controle Potencia Droop/6(Q)
  Vq/1 -> Sum5/1
  [Pref] -> P_Ref/1
  [Qref] -> Q_Ref/1
  [P3f] -> P/1
  [Sys_w] -> Imp. Virtual1/3(W)
  [Sw] -> Controle wt2/4(Sw)
  [Sys_wt] -> Controle wt2/1(Sys_wt)
  Controle Potencia Droop/2(Wref) -> Controle wt2/3(w_ref), [W0]
  [Vsd] -> Controle de potência modo conectado/3(Vsd)
  [Vsq] -> Controle de potência modo conectado/4(Vsq)
  [Sys_w] -> Controle wt2/2(Sys_w)
  LPF1/1 -> [P3f]
  LPF2/1 -> [Q3f]
  Medidor de pot/2(Q) -> LPF2/1
  [Iabc_M] -> PLL e Medidor1/1(Iabc_M)
  [Iabc_S] -> PLL e Medidor1/2(Iabc_S)
  Controle Potencia Droop/1(Vref) -> Sum4/1
  Imp. Virtual1/1(Vd_Zv) -> Sum4/2
  Imp. Virtual1/2(Vq_Zv) -> Sum5/2
  Controle wt2/1(wt) -> [wt]
  [wt] -> dq0 to abc1/2
  dq0 to abc1/1 -> Inversor CC/CA/1(Vabc)
  Referencia de  Corrente/2(Iq_ref) -> [Iqref]
  [Id_sup] -> Referencia de  Corrente/4(Id_supp)
  [Id] -> Controle Corrente/5(Id), Medidor de pot/3(Id)
  [Vabc_S] -> PLL e Medidor1/3(Vabc_S)
  [Vsd] -> Controle Corrente/3(Vsd), Controle de Tensao/5(Vsd), Medidor de pot/1(Vd)
  [Vsq] -> Controle Corrente/4(Vsq), Medidor de pot/2(Vq), Controle de Tensao/6(Vsq)
  Controle Corrente/2(Mq) -> [Mq]
  Medidor de pot/1(P) -> LPF1/1
  [Q3f] -> Mux2/3  "Q"
  [W0] -> W0/1, Mux2/6
  Mux3/1 -> Mux2/7
  Mux2/1 -> Reshape1/1
  Reshape1/1 -> Dados_Bat1/1
  [absV] -> Mux2/4  "V"
  [Pbat] -> Mux2/11
  [P3f] -> Mux2/1  "P"
  [absI] -> Mux2/5  "I"
  [Vbat] -> Mux2/10
  [Vdc] -> Mux2/8
  [Pref] -> Mux3/1
  [Sys_w] -> Wbat/1, Mux2/2
  [Qref] -> Mux3/2
  [Ibat] -> Mux2/9
  Elo CC/1(Vdc) -> Controle Tensao CC1/1(Vdc), Goto12/1
  Bateria e Conversor CC/CC1/2(Vbat) -> Goto13/1, Controle Tensao CC1/2(Vbat)
  Bateria e Conversor CC/CC1/1(Ibat) -> Goto11/1, Controle Tensao CC1/3(Ibat)
  Bateria e Conversor CC/CC1/3(Pbat) -> Goto14/1
  Controle Tensao CC1/1(D) -> Bateria e Conversor CC/CC1/1(D)
  Unit Delay1/1 -> dq0 to abc1/1
  Constant/1 -> Controle Corrente/8(Vdc)
  connections:
  Gnd1/RConn1 -- Inversor CC/CA/RConn4
  V&I - VSC2 1/RConn3 -- Vc1/RConn1
  Inversor CC/CA/RConn2 -- V&I - VSC2 1/LConn2
  V&I - VSC2 1/RConn1 -- Va1/RConn1
  V&I - VSC2 1/LConn1 -- Inversor CC/CA/RConn1
  V&I - VSC2 1/LConn3 -- Inversor CC/CA/RConn3
  V&I - VSC2 1/RConn2 -- Vb1/RConn1
  DC Voltage Source/LConn1 -- Inversor CC/CA/LConn2
  DC Voltage Source/RConn1 -- Inversor CC/CA/LConn1
  Elo CC/LConn1 -- Bateria e Conversor CC/CC1/LConn1
  Elo CC/LConn2 -- Bateria e Conversor CC/CC1/LConn2

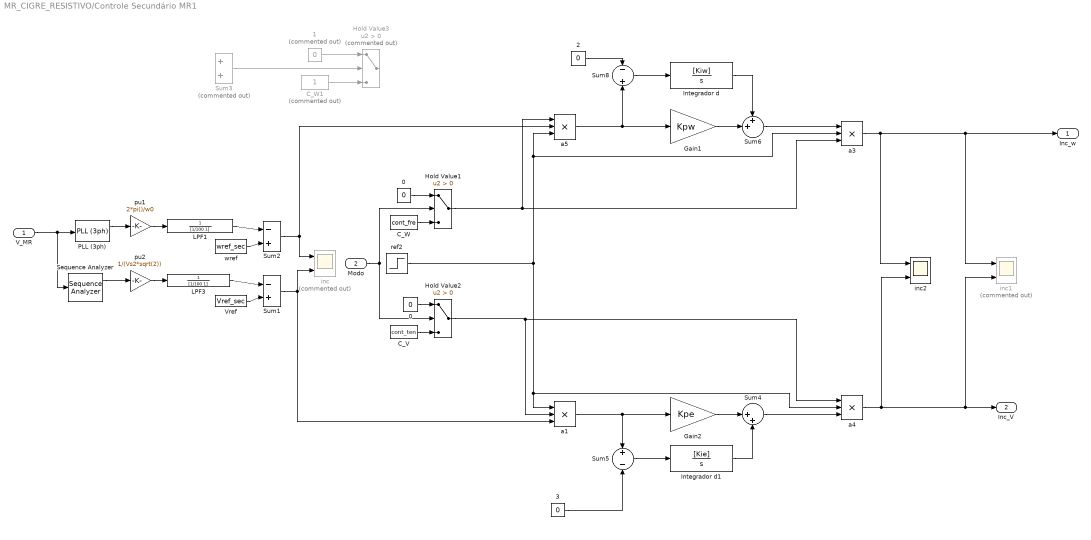
== system MR_CIGRE_RESISTIVO/Controle Secundário MR1 ==
  V_MR : Inport
  Modo : Inport  Port=2
  " 0 " : Constant  Value=0
  0 : Constant  Value=0
  1 : Constant  Commented=on  Value=0
  2 : Constant  Value=0
  3 : Constant  Value=0
  C_V : Constant  Value=cont_ten
  C_W : Constant  Value=cont_fre
  C_W1 : Constant  Commented=on
  Gain1 : Gain  Gain=Kpw
  Gain2 : Gain  Gain=Kpe
  Hold Value1 : Switch  Criteria=u2 > Threshold
  Hold Value2 : Switch  Criteria=u2 > Threshold
  Hold Value3 : Switch  Commented=on  Criteria=u2 > Threshold
  Integrador d : TransferFcn  Numerator=[Kiw]  Denominator=[1 0]
  Integrador d1 : TransferFcn  Numerator=[Kie]  Denominator=[1 0]
  LPF1 : TransferFcn  Denominator=[1/100 1]
  LPF3 : TransferFcn  Denominator=[1/100 1]
  PLL (3ph) : powerlib_meascontrol/PLL/PLL (3ph)  Fmin=1  Par_Init="[-0.57  f0]"  ParK=[180, 3200, 1]  TcD=5E-5  MaxRateChangeFreq=120  FilterCutOffFreq=25  Ts=5E-5  AGC=on
  Sequence Analyzer : powerlib_meascontrol/Measurements/Sequence Analyzer  Freq=50  n=1  seq=Positive  InInit=[1, 0]  Ts=0
      settings: SourceProductName=Simscape Power Systems  SourceProductBaseCode=PS
  Sum1 : Sum  Inputs=-|+
  Sum2 : Sum  Inputs=-|+
  Sum3 : Sum  Commented=on  Inputs=+|+
  Sum4 : Sum  Inputs=|++
  Sum5 : Sum  Inputs=+-
  Sum6 : Sum  Inputs=++|
  Sum8 : Sum  Inputs=-+
  Vref : Constant  Value=Vref_sec
  a{1,3..5} (4 alike) : Product  Inputs=***
  inc : Scope  Commented=on  NumInputPorts=2
  inc1 : Scope  Commented=on  NumInputPorts=2
  inc2 : Scope  NumInputPorts=2
  pu1 : Gain  Gain=2*pi()/w0
  pu2 : Gain  Gain=1/(Vs2*sqrt(2))
  ref2 : Step  Time=t_CS_ini  SampleTime=0
  wref : Constant  Value=wref_sec
  Inc_w : Outport
  Inc_V : Outport  Port=2
  wires:
  V_MR/1 -> Sequence Analyzer/1, PLL (3ph)/1
  pu2/1 -> LPF3/1
  Sum2/1 -> a5/2, inc/1
  LPF3/1 -> Sum1/1
  PLL (3ph)/1 -> pu1/1
  Sequence Analyzer/1 -> pu2/1
  Sum1/1 -> a1/3, inc/2
  pu1/1 -> LPF1/1
  LPF1/1 -> Sum2/1
  wref/1 -> Sum2/2
  Hold Value1/1 -> a3/3, a5/1
  Sum6/1 -> a3/1
  Vref/1 -> Sum1/2
  Hold Value2/1 -> a4/1, a1/2
  Modo/1 -> Hold Value1/2, Hold Value2/2
  ref2/1 -> a4/2, a1/1, a3/2, a5/3
  C_W/1 -> Hold Value1/3
  0/1 -> Hold Value1/1
  " 0 "/1 -> Hold Value2/1
  C_V/1 -> Hold Value2/3
  Sum3/1 -> Hold Value3/2
  ? -> Sum3/1
  ? -> Sum3/2
  1/1 -> Hold Value3/1
  Integrador d/1 -> Sum6/1
  Gain1/1 -> Sum6/2
  a5/1 -> Sum8/2, Gain1/1
  a1/1 -> Gain2/1, Sum5/1
  Gain2/1 -> Sum4/1
  Integrador d1/1 -> Sum4/2
  Sum4/1 -> a4/3
  Sum5/1 -> Integrador d1/1
  Sum8/1 -> Integrador d/1
  C_W1/1 -> Hold Value3/3
  3/1 -> Sum5/2
  a3/1 -> inc1/1, Inc_w/1, inc2/1
  a4/1 -> inc1/2, Inc_V/1, inc2/2
  2/1 -> Sum8/1

== system MR_CIGRE_RESISTIVO/Mundaça Modo Fonte VF ==
  sinc : Inport
  BAT1 : Switch  Criteria=u2 > Threshold
  BAT1_CONT : Constant  Value=BAT1_CONT
  BAT2 : Switch  Criteria=u2 > Threshold
  BAT2_CONT : Constant  Value=BAT2_CONT
  Conectado Ilhado Conectado1 : Switch  Criteria=u2 > Threshold
  PQ : Constant
  PQ para Vf : Step  Time=tilha+t_atraso  Before=1  After=0  SampleTime=0
  Bat1 : Outport
  Bat2 : Outport  Port=2
  Fonte : Outport  Port=3
  wires:
  sinc/1 -> Conectado Ilhado Conectado1/2
  PQ para Vf/1 -> Conectado Ilhado Conectado1/3
  Conectado Ilhado Conectado1/1 -> Fonte/1, BAT2/3, BAT1/3
  PQ/1 -> Conectado Ilhado Conectado1/1, BAT2/1, BAT1/1
  BAT1_CONT/1 -> BAT1/2
  BAT1/1 -> Bat1/1
  BAT2/1 -> Bat2/1
  BAT2_CONT/1 -> BAT2/2

== system MR_CIGRE_RESISTIVO/PCC ==
  sinc : Inport
  Dados_PCC : ToWorkspace  VariableName=PCC  SampleTime=-1
  Gain1 : Gain  Gain=-1
  Gain5 : Gain  Gain=-1
  Ilhamento/ Sincronização : Subsystem
  Mux4 : Mux
  "PCC Se ch =1, chave fechada Se ch =0, chave aberta" : powerlib/Elements/Three-Phase Breaker  InitialState=closed  SwitchA=on  SwitchB=on  SwitchC=on  SwitchTimes=[tilha tilha+1]  External=on  BreakerResistance=0.01  SnubberResistance=1e5  SnubberCapacitance=inf  Measurements=None
      settings: AttributesFormatString=\n
  PCC_MED : powerlib/Measurements/Three-Phase V-I Measurement  VoltageMeasurement=phase-to-ground  SetLabelV=off  LabelV=Vabc  Vpu=off  VpuLL=off  CurrentMeasurement=yes  SetLabelI=off  LabelI=Iabc  Ipu=off  Pbase=Sb  Vbase=Vs2  OutputType=Complex  PhasorSimulation=off  PSBequivalent=0
  PLL (3ph) : powerlib_meascontrol/PLL/PLL (3ph)  Commented=on  Fmin=45  Par_Init=[0, 60]  ParK=[180, 3200, 1]  TcD=1e-4  MaxRateChangeFreq=200  FilterCutOffFreq=25  Ts=0  AGC=on
  Power : powerlib_meascontrol/Measurements/Power (Positive-Sequence)  Freq=f0  Vinit=[0, 0]  Iinit=[0, 0]  Ts=0
      settings: SourceProductName=Simscape Power Systems  SourceProductBaseCode=PS
  Sequence Analyzer : powerlib_meascontrol/Measurements/Sequence Analyzer  Freq=f0  n=1  seq=Positive  InInit=[1, 0]  Ts=0
      settings: SourceProductName=Simscape Power Systems  SourceProductBaseCode=PS
  A : PMIOPort  Port=1  Side=Left
  B : PMIOPort  Port=2  Side=Left
  C : PMIOPort  Port=3  Side=Left
  A_out : PMIOPort  Port=4  Side=Right
  B_out : PMIOPort  Port=5  Side=Right
  C_out : PMIOPort  Port=6  Side=Right
  P : Outport
  Q : Outport  Port=2
  V : Outport  Port=3
  f : Outport  Port=4
  wires:
  PLL (3ph)/1 -> Mux4/4, f/1
  Power/1 -> Gain5/1
  Power/2 -> Gain1/1
  PCC_MED/2 -> Power/2
  sinc/1 -> Ilhamento/ Sincronização/1(sinc)
  PCC_MED/1 -> Power/1, Sequence Analyzer/1, PLL (3ph)/1
  Sequence Analyzer/1 -> Mux4/3, V/1
  Ilhamento/ Sincronização/1("Ch ") -> "PCC Se ch =1, chave fechada Se ch =0, chave aberta"/1
  Gain5/1 -> Mux4/1, P/1
  Gain1/1 -> Mux4/2, Q/1
  Mux4/1 -> Dados_PCC/1
  connections:
  "PCC Se ch =1, chave fechada Se ch =0, chave aberta"/RConn3 -- PCC_MED/RConn3
  "PCC Se ch =1, chave fechada Se ch =0, chave aberta"/RConn1 -- PCC_MED/RConn1
  PCC_MED/LConn1 -- A_out/RConn1
  "PCC Se ch =1, chave fechada Se ch =0, chave aberta"/RConn2 -- PCC_MED/RConn2
  PCC_MED/LConn2 -- B_out/RConn1
  PCC_MED/LConn3 -- C_out/RConn1
  C/RConn1 -- "PCC Se ch =1, chave fechada Se ch =0, chave aberta"/LConn3
  B/RConn1 -- "PCC Se ch =1, chave fechada Se ch =0, chave aberta"/LConn2
  A/RConn1 -- "PCC Se ch =1, chave fechada Se ch =0, chave aberta"/LConn1

== system MR_CIGRE_RESISTIVO/R1 ==
  1/Ib : Gain  Gain=(1)/(sqrt(2))
  1/Vb : Gain  Gain=sqrt(3)/(1*sqrt(2))
  BCarga : powerlib/Measurements/Three-Phase V-I Measurement  VoltageMeasurement=phase-to-ground  SetLabelV=off  LabelV=Vabc_B2  Vpu=off  VpuLL=off  CurrentMeasurement=yes  SetLabelI=off  LabelI=Iabc_B120  Ipu=off  Pbase=100e6  Vbase=Vs2  OutputType=Complex  PhasorSimulation=off  PSBequivalent=0
  CCV1 : powerlib/Elements/Three-Phase Breaker  Commented=on  InitialState=open  SwitchA=on  SwitchB=on  SwitchC=on  SwitchTimes=[TLR11 TDR1]  External=off  BreakerResistance=0.01  SnubberResistance=1e5  SnubberCapacitance=inf  Measurements=None
      settings: AttributesFormatString=\n
  Carga Fixa : powerlib/Elements/Three-Phase Series RLC Load  LConnTagsString=A|B|C  Configuration=Y (grounded)  NominalVoltage=Vs2  Vabc=[1e3 1e3 1e3]  Vabcp=[1e3 1e3 1e3]  NominalFrequency=f0  UnbalancedPower=off  ActivePower=PLoadR1  InductivePower=QLoadR1  CapacitivePower=0  Pabc=[10e3 9e3 11e3]  QLabc=[100 90 110]  QCabc=[100 90 110]  Pabcp=[10e3 9e3 11e3]  QLabcp=[100 90 110]  QCabcp=[100 90 110]  Measurements=None  LoadType=constant Z
  Carga Variável : powerlib/Elements/Three-Phase Series RLC Load  Commented=on  LConnTagsString=A|B|C  Configuration=Y (grounded)  NominalVoltage=Vs2  Vabc=[1e3 1e3 1e3]  Vabcp=[1e3 1e3 1e3]  NominalFrequency=f0  UnbalancedPower=off  ActivePower=P_var_loadR1  InductivePower=Q_var_loadR1  CapacitivePower=0  Pabc=[10e3 9e3 11e3]  QLabc=[100 90 110]  QCabc=[100 90 110]  Pabcp=[10e3 9e3 11e3]  QLabcp=[100 90 110]  QCabcp=[100 90 110]  Measurements=None  LoadType=constant Z
  Dados_C1 : ToWorkspace  Commented=on  VariableName=R01  SaveFormat=Structure With Time  SampleTime=-1
  Ip : powerlib_meascontrol/Measurements/Sequence Analyzer  Freq=f0  n=1  seq=Positive  InInit=[1, 0]  Ts=0
      settings: SourceProductName=Simscape Power Systems  SourceProductBaseCode=PS
  Mux9 : Mux  Commented=on
  Power : powerlib_meascontrol/Measurements/Power (Positive-Sequence)  Freq=f0  Vinit=[0, 0]  Iinit=[0, 0]  Ts=0
      settings: SourceProductName=Simscape Power Systems  SourceProductBaseCode=PS
  Reshape : Reshape  Commented=on  OutputDimensions=[1,7]
  Vp : powerlib_meascontrol/Measurements/Sequence Analyzer  Freq=f0  n=1  seq=Positive  InInit=[1, 0]  Ts=0
      settings: SourceProductName=Simscape Power Systems  SourceProductBaseCode=PS
  fa : PMIOPort  Port=1  Side=Left
  fb : PMIOPort  Port=2  Side=Left
  fc : PMIOPort  Port=3  Side=Left
  P : Outport
  V : Outport  Port=2
  Q : Outport  Port=3
  I : Outport  Port=4
  wires:
  BCarga/1 -> Power/1, Vp/1
  Mux9/1 -> Reshape/1
  BCarga/2 -> Power/2, Ip/1
  Power/1 -> Mux9/1, P/1
  1/Vb/1 -> V/1, Mux9/2
  1/Ib/1 -> I/1, Mux9/4
  Vp/1 -> 1/Vb/1
  Ip/1 -> 1/Ib/1
  Power/2 -> Q/1, Mux9/3
  Reshape/1 -> Dados_C1/1
  connections:
  BCarga/LConn3 -- fc/RConn1
  BCarga/LConn2 -- fb/RConn1
  BCarga/LConn1 -- fa/RConn1
  BCarga/RConn3 -- CCV1/RConn3 -- Carga Fixa/LConn3
  BCarga/RConn1 -- CCV1/RConn1 -- Carga Fixa/LConn1
  BCarga/RConn2 -- CCV1/RConn2 -- Carga Fixa/LConn2
  CCV1/LConn1 -- Carga Variável/LConn1
  CCV1/LConn3 -- Carga Variável/LConn3
  CCV1/LConn2 -- Carga Variável/LConn2

== system MR_CIGRE_RESISTIVO/R1-R2 ==
  1 : powerlib/Elements/Series RLC Branch  LConnTagsString=__new0  RConnTagsString=__new0  BranchType=RL  Resistance=R_1_2  Inductance=L_1_2  SetiL0=off  InitialCurrent=0  Capacitance=1e-6  Setx0=off  InitialVoltage=0  Measurements=None
  2 : powerlib/Elements/Series RLC Branch  LConnTagsString=__new0  RConnTagsString=__new0  BranchType=RL  Resistance=R_1_2  Inductance=L_1_2  SetiL0=off  InitialCurrent=0  Capacitance=1e-6  Setx0=off  InitialVoltage=0  Measurements=None
  3 : powerlib/Elements/Series RLC Branch  LConnTagsString=__new0  RConnTagsString=__new0  BranchType=RL  Resistance=R_1_2  Inductance=L_1_2  SetiL0=off  InitialCurrent=0  Capacitance=1e-6  Setx0=off  InitialVoltage=0  Measurements=None
  A : PMIOPort  Port=1  Side=Left
  a : PMIOPort  Port=2  Side=Right
  B : PMIOPort  Port=3  Side=Left
  b : PMIOPort  Port=4  Side=Right
  C : PMIOPort  Port=5  Side=Left
  c : PMIOPort  Port=6  Side=Right
  connections:
  1/LConn1 -- A/RConn1
  2/LConn1 -- B/RConn1
  3/LConn1 -- C/RConn1
  1/RConn1 -- a/RConn1
  2/RConn1 -- b/RConn1
  3/RConn1 -- c/RConn1

== system MR_CIGRE_RESISTIVO/R10_R18 ==
  1 : powerlib/Elements/Series RLC Branch  LConnTagsString=__new0  RConnTagsString=__new0  BranchType=RL  Resistance=R_10_18  Inductance=L_10_18  SetiL0=off  InitialCurrent=0  Capacitance=1e-6  Setx0=off  InitialVoltage=0  Measurements=None
  2 : powerlib/Elements/Series RLC Branch  LConnTagsString=__new0  RConnTagsString=__new0  BranchType=RL  Resistance=R_10_18  Inductance=L_10_18  SetiL0=off  InitialCurrent=0  Capacitance=1e-6  Setx0=off  InitialVoltage=0  Measurements=None
  3 : powerlib/Elements/Series RLC Branch  LConnTagsString=__new0  RConnTagsString=__new0  BranchType=RL  Resistance=R_10_18  Inductance=L_10_18  SetiL0=off  InitialCurrent=0  Capacitance=1e-6  Setx0=off  InitialVoltage=0  Measurements=None
  A : PMIOPort  Port=1  Side=Left
  a : PMIOPort  Port=2  Side=Right
  B : PMIOPort  Port=3  Side=Left
  b : PMIOPort  Port=4  Side=Right
  C : PMIOPort  Port=5  Side=Left
  c : PMIOPort  Port=6  Side=Right
  connections:
  1/LConn1 -- A/RConn1
  2/LConn1 -- B/RConn1
  3/LConn1 -- C/RConn1
  1/RConn1 -- a/RConn1
  2/RConn1 -- b/RConn1
  3/RConn1 -- c/RConn1
